simulink model "simulink_control"  (R2025b)
settings: Solver=ode4  StartTime=0.0  StopTime=inf  FixedStep=0.016  RelTol=1e-3
values from neighbouring files (symbols this model uses):
  accelerometer_sensor = wb_robot_get_device('accelerometer')    [simulink_control_app.m]
  alpha_pitch = 0.85    [simulink_control_app.m]
  gps_sensor = wb_robot_get_device('gps')    [simulink_control_app.m]
  gyro_sensor = wb_robot_get_device('gyro')    [simulink_control_app.m]
  inertial_unit = wb_robot_get_device('inertial_unit')    [simulink_control_app.m]
  left_trushter_motor = wb_robot_get_device('left_motor')    [simulink_control_app.m]
  right_trushter_motor = wb_robot_get_device('right_motor')    [simulink_control_app.m]
  TIME_STEP = 16    [simulink_control_app.m]
undefined symbols (not defined in the file or in its folder): gray, mission_waypoints
libraries: simulink_extras x5, eeGeneralControl x2
settings Model: Creator=Harun  LastModifiedBy=Szymon
settings DebuggingCC: UnderSpecifiedDimensionMsg=warning

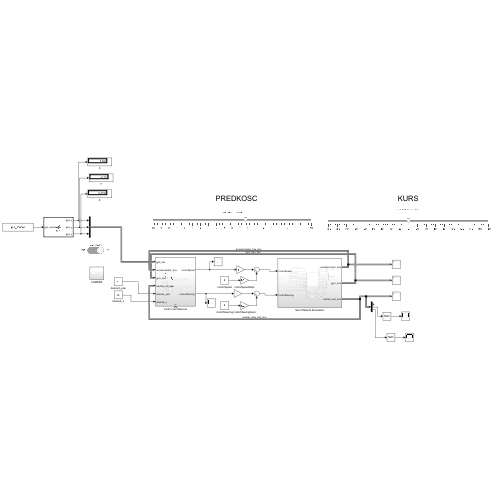
[thumbnail: Simulink's stored preview of the top-level diagram]
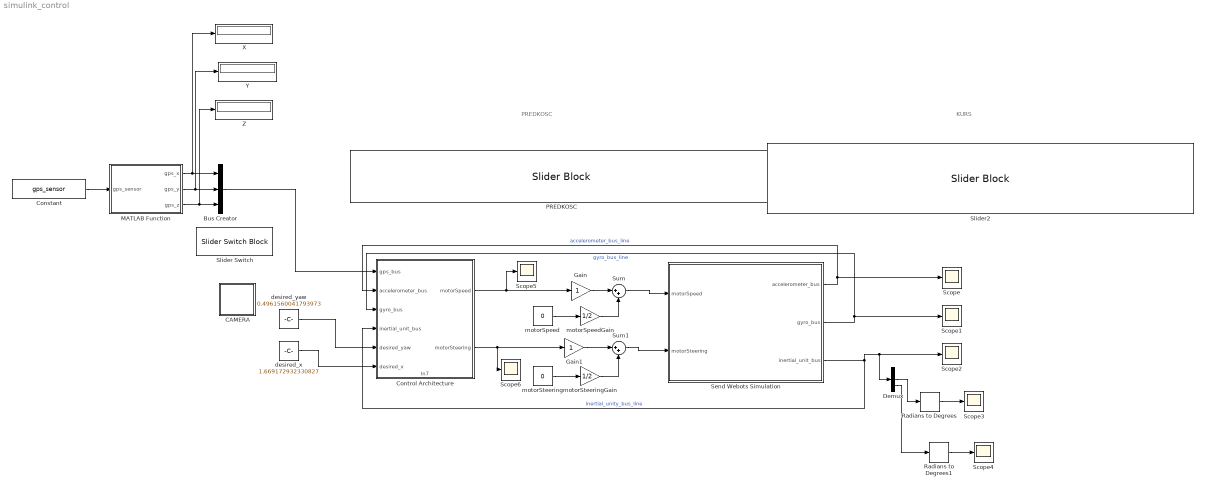
== system simulink_control ==
  note: KURS
  note: PREDKOSC
  Bus Creator : BusCreator  Inputs=3
  CAMERA : Subsystem
  Constant : Constant  Value=gps_sensor
  Control Architecture : Subsystem
      settings: PortSchema="{\"entries\":[{\"content\":{\"sides\":[{\"content\":{\"connectorIds\":[\"In1\",\"In2\",\"In3\",\"In4\",\"In5\",\"In6\"]},\"type\":\"ConnectorPlacement.EquallySpacedRectSide\",\"uuid\":\"94cabca2-e76e-4691-9816-b95fb886a2a7\"},{\"content\":{\"connectorIds\":[\"Out1\",\"Out2\"],\"side\":\"RIGHT\"},\"type\":\"ConnectorPlacement.EquallySpacedRectSide\",\"uuid\":\"240d2e1d-620c-4ca0-9643-bfc077ee6341\"},{\"content\":{\"side\":\"TOP\"},\"type\":\"ConnectorPlacement.EquallySpacedRectSide\",\"uuid\":\"858b813a-0718-4a6f-97d6-2c7be5dc6086\"},{\"content\":{\"connectorIds\":[\"In7\"],\"side\":\"BOTTOM\"},\"type\":\"ConnectorPlacement.EquallySpacedRectSide\",\"uuid\":\"e25d5035-11e6-4256-b3cd-0a1c699f2cde\"}]},\"type\":\"ConnectorPlacement.EquallySpacedConnector\",\"uuid\":\"155b933b-e855-4e90-a0aa-f79b0a1ce075\"}],\"packageUris\":[\"http://schema.mathworks.com/mf0/Connector/R2020b\"],\"version\":\"1.0\"}"
  Demux : Demux  Outputs=3
  Gain : Gain
  Gain1 : Gain
  MATLAB Function : MATLAB Function  TreatAsAtomicUnit=on
  PREDKOSC : SliderBlock  ScaleMin=-10  ScaleMax=10
  Radians to Degrees : simulink_extras/Transformations/Radians to Degrees
  Radians to Degrees1 : simulink_extras/Transformations/Radians to Degrees
  Scope{,1..6} (7 alike) : Scope
      Scope settings: ActiveDisplayYMinimum=-30.6391  ActiveDisplayYMaximum=29.79687
      Scope1 settings: ActiveDisplayYMinimum=-12220.56497  ActiveDisplayYMaximum=12217.33322
      Scope2 settings: ActiveDisplayYMinimum=-3.8392  ActiveDisplayYMaximum=3.73806
      Scope3 settings: ActiveDisplayYMinimum=-1.49091  ActiveDisplayYMaximum=-1.14094  DataLoggingVariableName=ScopeData2
      Scope4 settings: ActiveDisplayYMinimum=-48.59786  ActiveDisplayYMaximum=-34.20452  DataLoggingVariableName=ScopeData2
      Scope5 settings: ActiveDisplayYMinimum=-0.00358  ActiveDisplayYMaximum=0.03222  DataLoggingVariableName=ScopeData5
      Scope6 settings: ActiveDisplayYMinimum=-0.15563  ActiveDisplayYMaximum=1.4007  DataLoggingVariableName=ScopeData2
  Send Webots Simulation : Subsystem
  Slider Switch : SliderSwitchBlock
  Slider2 : SliderBlock  ScaleMin=-180  ScaleMax=180  TickInterval=20
  Sum : Sum  Inputs=|++
  Sum1 : Sum  Inputs=|++
  X : Display
  Y : Display
  Z : Display
  desired_x : Constant  Value=1.669172932330827
  desired_yaw : Constant  Value=0.4961560041793973
  motorSpeed : Constant  Value=0
  motorSpeedGain : Gain  Gain=1/2
  motorSteering : Constant  Value=0
  motorSteeringGain : Gain  Gain=1/2
  wires:
  motorSteering/1 -> motorSteeringGain/1
  motorSpeed/1 -> motorSpeedGain/1
  Sum/1 -> Send Webots Simulation/1(motorSpeed)
  Control Architecture/1(motorSpeed) -> Scope5/1, Gain/1
  Control Architecture/2(motorSteering) -> Scope6/1, Gain1/1
  Sum1/1 -> Send Webots Simulation/2(motorSteering)
  motorSpeedGain/1 -> Sum/2
  motorSteeringGain/1 -> Sum1/2
  Send Webots Simulation/1(accelerometer_bus) -> Control Architecture/2(accelerometer_bus), Scope/1  "accelerometer_bus_line"
  Send Webots Simulation/2(gyro_bus) -> Control Architecture/3(gyro_bus), Scope1/1  "gyro_bus_line"
  Send Webots Simulation/3(inertial_unit_bus) -> Demux/1, Scope2/1, Control Architecture/4(inertial_unit_bus)  "inertial_unity_bus_line"
  Gain/1 -> Sum/1
  Demux/2 -> Radians to Degrees/1
  Radians to Degrees/1 -> Scope3/1
  Radians to Degrees1/1 -> Scope4/1
  Demux/3 -> Radians to Degrees1/1
  Gain1/1 -> Sum1/1
  desired_x/1 -> Control Architecture/6(desired_x)
  desired_yaw/1 -> Control Architecture/5(desired_yaw)
  Constant/1 -> MATLAB Function/1(gps_sensor)
  MATLAB Function/2(gps_y) -> Y/1, Bus Creator/2
  MATLAB Function/3(gps_z) -> Z/1, Bus Creator/3
  MATLAB Function/1(gps_x) -> X/1, Bus Creator/1
  Bus Creator/1 -> Control Architecture/1(gps_bus)

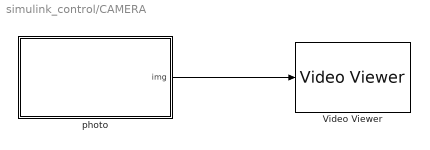
== system simulink_control/CAMERA ==
  Video Viewer : VideoViewer  colormapValue=gray(256)  FigPos=[1 1158 1920 1061]
  photo : MATLAB Function  TreatAsAtomicUnit=on
  wires:
  photo/1(img) -> Video Viewer/1

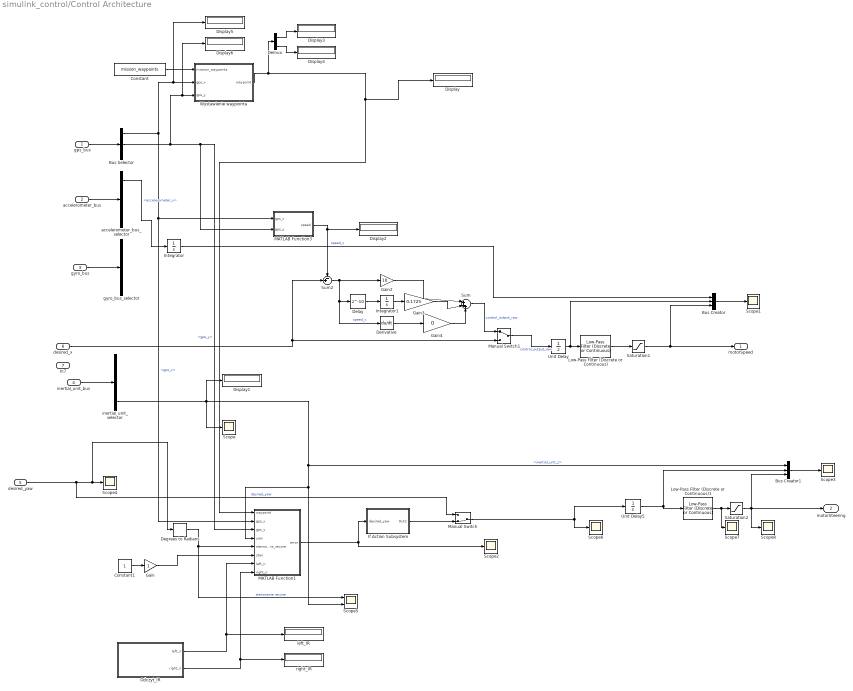
== system simulink_control/Control Architecture ==
  gps_bus : Inport
  accelerometer_bus : Inport  Port=2
  gyro_bus : Inport  Port=3
  inertial_unit_bus : Inport  Port=4
  desired_yaw : Inport  Port=5
  desired_x : Inport  Port=6
  In7 : Inport  Port=7
  Bus Creator : BusCreator  Inputs=3
  Bus Creator1 : BusCreator  Inputs=3
  Bus Selector : BusSelector  OutputSignals=gps_x,gps_y,gps_z
  Constant : Constant  Value=mission_waypoints
  Constant1 : Constant
  Degrees to Radians : simulink_extras/Transformations/Degrees to Radians
  Delay : Delay  DelayLength=10
  Demux : Demux  Outputs=2
  Derivative : Derivative  CoefficientInTFapproximation=0.016
  Display{,1..6} (7 alike) : Display
  Gain : Gain
  Gain2 : Gain  Gain=10
  Gain3 : Gain  Gain=0.1725
  Gain4 : Gain  Gain=0
  If Action Subsystem : Subsystem  TreatAsAtomicUnit=on
  Integrator : Integrator
  Integrator1 : Integrator
  Low-Pass Filter (Discrete or Continuous) : eeGeneralControl/Low-Pass Filter (Discrete or Continuous)  K=1  T=0.016  B=inf  A=-inf  init_option=Inherited from block input  x0=0  Ts=-1
  Low-Pass Filter (Discrete or Continuous)1 : eeGeneralControl/Low-Pass Filter (Discrete or Continuous)  K=1  T=0.016  B=inf  A=-inf  init_option=Inherited from block input  x0=0  Ts=-1
  MATLAB Function1 : MATLAB Function  TreatAsAtomicUnit=on
  MATLAB Function3 : MATLAB Function  TreatAsAtomicUnit=on
  Manual Switch : ManualSwitch  CurrentSetting=0
  Manual Switch1 : ManualSwitch
  Odczyt_IR : MATLAB Function  TreatAsAtomicUnit=on
  Saturation1 : Saturate  UpperLimit=15  LowerLimit=-15
  Saturation2 : Saturate  UpperLimit=5  LowerLimit=-5
  Scope{,1..4,6..8} (8 alike) : Scope
      Scope settings: ActiveDisplayYMinimum=-0.84582  ActiveDisplayYMaximum=3.34904
      Scope1 settings: ActiveDisplayYMinimum=-78.38231  ActiveDisplayYMaximum=106.01245  DataLoggingVariableName=ScopeData2
      Scope2 settings: ActiveDisplayYMinimum=-0.00316  ActiveDisplayYMaximum=0.00341  DataLoggingVariableName=ScopeData3
      Scope3 settings: ActiveDisplayYMinimum=-48028.32937  ActiveDisplayYMaximum=47920.10481
      Scope4 settings: ActiveDisplayYMinimum=85.82399  ActiveDisplayYMaximum=105.82399
      Scope6 settings: ActiveDisplayYMinimum=-1006.23593  ActiveDisplayYMaximum=1051.55838  DataLoggingVariableName=ScopeData3
      Scope7 settings: ActiveDisplayYMinimum=-7.95026  ActiveDisplayYMaximum=65.1796  DataLoggingVariableName=ScopeData4
      Scope8 settings: ActiveDisplayYMinimum=-0.15563  ActiveDisplayYMaximum=1.4007  DataLoggingVariableName=ScopeData5
  Scope5 : Scope  NumInputPorts=2
      settings: ActiveDisplayYMinimum=-3.49256  ActiveDisplayYMaximum=3.48254  DataLoggingVariableName=ScopeData2
  Sum : Sum  Inputs=|+++
  Sum2 : Sum  Inputs=-+|
  Unit Delay : UnitDelay  SampleTime=-1  HasFrameUpgradeWarning=on
  Unit Delay5 : UnitDelay  SampleTime=-1  HasFrameUpgradeWarning=on
  Wystawienie waypointa : MATLAB Function  TreatAsAtomicUnit=on
  accelerometer_bus_selector : BusSelector  OutputSignals=accelerometer_x,accelerometer_y,accelerometer_z
  gyro_bus_selector : BusSelector  OutputSignals=gyro_x,gyro_y,gyro_z
  inertial_unit_selector : BusSelector  OutputSignals=inertial_unit_x,inertial_unit_y,inertial_unit_z
  left_IR : Display
  right_IR : Display
  motorSpeed : Outport
  motorSteering : Outport  Port=2
  wires:
  accelerometer_bus/1 -> accelerometer_bus_selector/1
  gyro_bus/1 -> gyro_bus_selector/1
  inertial_unit_bus/1 -> inertial_unit_selector/1
  Bus Creator/1 -> Scope1/1
  inertial_unit_selector/3 -> Scope/1, Display1/1, Scope5/2, MATLAB Function1/4(yaw), Bus Creator1/1  "<inertial_unit_z>"
  Saturation1/1 -> motorSpeed/1, Bus Creator/3
  Integrator/1 -> Bus Creator/1  "speed_x"
  Unit Delay/1 -> Bus Creator/2, Low-Pass Filter (Discrete or Continuous)/1
  Low-Pass Filter (Discrete or Continuous)/1 -> Saturation1/1
  Unit Delay5/1 -> Low-Pass Filter (Discrete or Continuous)1/1, Bus Creator1/2
  Bus Creator1/1 -> Scope3/1
  accelerometer_bus_selector/1 -> Integrator/1  "<accelerometer_x>"
  gps_bus/1 -> Bus Selector/1
  Bus Selector/1 -> MATLAB Function1/2(gps_x), MATLAB Function3/1(gps_x), Display5/1, Wystawienie waypointa/2(gps_x)  "<gps_x>"
  Bus Selector/2 -> MATLAB Function3/2(gps_y), MATLAB Function1/3(gps_y), Display6/1, Wystawienie waypointa/3(gps_y)  "<gps_y>"
  Manual Switch/1 -> Unit Delay5/1, Scope6/1
  desired_yaw/1 -> Manual Switch/1, Scope4/1, Degrees to Radians/1  "desired_yaw"
  Saturation2/1 -> Scope8/1, motorSteering/1, Bus Creator1/3
  Degrees to Radians/1 -> Scope5/1, MATLAB Function1/5(sterwowanie_reczne)  "sterowanie reczne"
  Low-Pass Filter (Discrete or Continuous)1/1 -> Scope7/1, Saturation2/1
  Wystawienie waypointa/1(waypoint) -> MATLAB Function1/1(waypoint), Display/1, Demux/1
  MATLAB Function3/1(speed) -> Sum2/1, Display2/1
  desired_x/1 -> Sum2/2, Manual Switch1/2
  Sum2/1 -> Gain2/1, Derivative/1, Delay/1  "speed_x"
  Manual Switch1/1 -> Unit Delay/1  "control_output_raw"
  Integrator1/1 -> Gain3/1
  Gain3/1 -> Sum/2
  Gain2/1 -> Sum/1
  Derivative/1 -> Gain4/1
  Gain4/1 -> Sum/3
  Sum/1 -> Manual Switch1/1  "control_output_raw"
  MATLAB Function1/1(error) -> Scope2/1, If Action Subsystem/1(desired_yaw)
  If Action Subsystem/1(Out2) -> Manual Switch/2
  Delay/1 -> Integrator1/1
  Demux/1 -> Display3/1
  Demux/2 -> Display4/1
  Constant/1 -> Wystawienie waypointa/1(mission_waypoints)
  Gain/1 -> MATLAB Function1/6(stan)
  Constant1/1 -> Gain/1
  Odczyt_IR/1(left_ir) -> MATLAB Function1/7(left_ir), left_IR/1
  Odczyt_IR/2(right_ir) -> MATLAB Function1/8(right_ir), right_IR/1

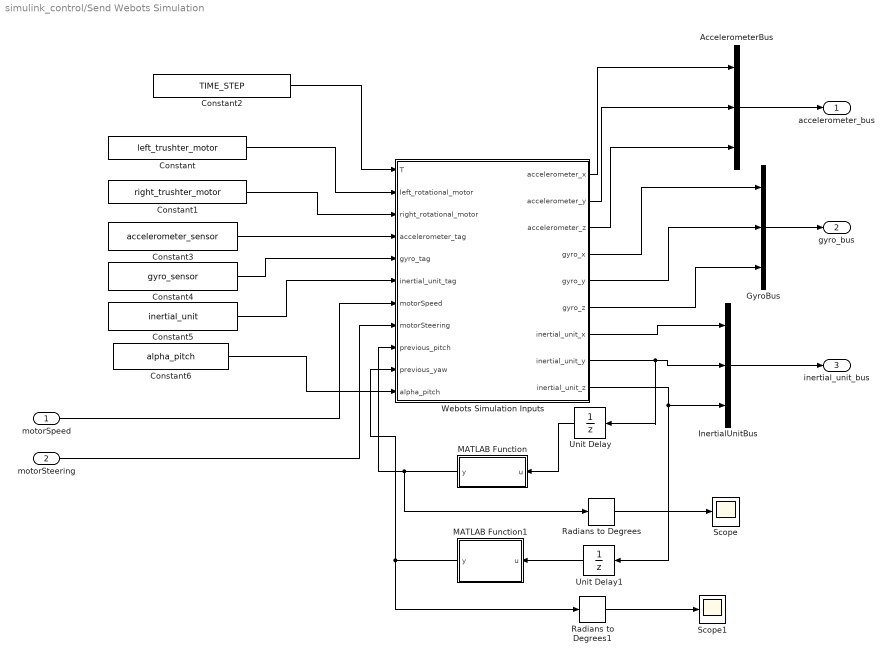
== system simulink_control/Send Webots Simulation ==
  motorSpeed : Inport
  motorSteering : Inport  Port=2
  AccelerometerBus : BusCreator  Inputs=3
  Constant : Constant  Value=left_trushter_motor
  Constant1 : Constant  Value=right_trushter_motor
  Constant2 : Constant  Value=TIME_STEP
  Constant3 : Constant  Value=accelerometer_sensor
  Constant4 : Constant  Value=gyro_sensor
  Constant5 : Constant  Value=inertial_unit
  Constant6 : Constant  Value=alpha_pitch
  GyroBus : BusCreator  Inputs=3
  InertialUnitBus : BusCreator  Inputs=3
  MATLAB Function : MATLAB Function  TreatAsAtomicUnit=on
  MATLAB Function1 : MATLAB Function  TreatAsAtomicUnit=on
  Radians to Degrees : simulink_extras/Transformations/Radians to Degrees
  Radians to Degrees1 : simulink_extras/Transformations/Radians to Degrees
  Scope : Scope
      settings: ActiveDisplayYMinimum=-1.32337  ActiveDisplayYMaximum=0.14704
  Scope1 : Scope
      settings: ActiveDisplayYMinimum=-221.28069  ActiveDisplayYMaximum=223.17839  DataLoggingVariableName=ScopeData3
  Unit Delay : UnitDelay  SampleTime=-1  HasFrameUpgradeWarning=on
  Unit Delay1 : UnitDelay  SampleTime=-1  HasFrameUpgradeWarning=on
  Webots Simulation Inputs : MATLAB Function  TreatAsAtomicUnit=on
  accelerometer_bus : Outport
  gyro_bus : Outport  Port=2
  inertial_unit_bus : Outport  Port=3
  wires:
  motorSpeed/1 -> Webots Simulation Inputs/7(motorSpeed)
  Constant1/1 -> Webots Simulation Inputs/3(right_rotational_motor)
  Constant2/1 -> Webots Simulation Inputs/1(T)
  Constant/1 -> Webots Simulation Inputs/2(left_rotational_motor)
  Webots Simulation Inputs/2(accelerometer_y) -> AccelerometerBus/2
  Webots Simulation Inputs/1(accelerometer_x) -> AccelerometerBus/1
  Webots Simulation Inputs/3(accelerometer_z) -> AccelerometerBus/3
  AccelerometerBus/1 -> accelerometer_bus/1
  Constant3/1 -> Webots Simulation Inputs/4(accelerometer_tag)
  motorSteering/1 -> Webots Simulation Inputs/8(motorSteering)
  Constant4/1 -> Webots Simulation Inputs/5(gyro_tag)
  Webots Simulation Inputs/6(gyro_z) -> GyroBus/3
  Webots Simulation Inputs/5(gyro_y) -> GyroBus/2
  GyroBus/1 -> gyro_bus/1
  Webots Simulation Inputs/4(gyro_x) -> GyroBus/1
  Webots Simulation Inputs/7(inertial_unit_x) -> InertialUnitBus/1
  Webots Simulation Inputs/8(inertial_unit_y) -> Unit Delay/1, InertialUnitBus/2
  Webots Simulation Inputs/9(inertial_unit_z) -> Unit Delay1/1, InertialUnitBus/3
  InertialUnitBus/1 -> inertial_unit_bus/1
  Constant5/1 -> Webots Simulation Inputs/6(inertial_unit_tag)
  Constant6/1 -> Webots Simulation Inputs/11(alpha_pitch)
  MATLAB Function/1(y) -> Radians to Degrees/1, Webots Simulation Inputs/9(previous_pitch)
  Unit Delay/1 -> MATLAB Function/1(u)
  Radians to Degrees/1 -> Scope/1
  Unit Delay1/1 -> MATLAB Function1/1(u)
  Radians to Degrees1/1 -> Scope1/1
  MATLAB Function1/1(y) -> Radians to Degrees1/1, Webots Simulation Inputs/10(previous_yaw)

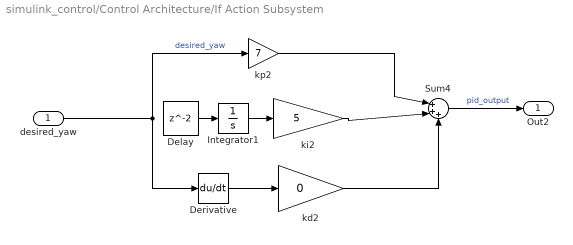
== system simulink_control/Control Architecture/If Action Subsystem ==
  desired_yaw : Inport
  Delay : Delay
  Derivative : Derivative
  Integrator1 : Integrator
  Sum4 : Sum  Inputs=|+++
  kd2 : Gain  Gain=0
  ki2 : Gain  Gain=5
  kp2 : Gain  Gain=7
  Out2 : Outport
  wires:
  Sum4/1 -> Out2/1  "pid_output"
  kp2/1 -> Sum4/1
  ki2/1 -> Sum4/2
  Integrator1/1 -> ki2/1
  desired_yaw/1 -> Derivative/1, kp2/1  "desired_yaw"
  kd2/1 -> Sum4/3
  Derivative/1 -> kd2/1
  Delay/1 -> Integrator1/1

== matlab function simulink_control/Control Architecture/MATLAB Function1 ==
  data: waypoint input; error output; gps_x input; gps_y input; yaw input; sterwowanie_reczne input; stan input; left_ir input; right_ir input
function error = guidance(waypoint, gps_x, gps_y, yaw, sterwowanie_reczne, stan, left_ir, right_ir)
persistent timer_ucieczki kat_ucieczki

if isempty(timer_ucieczki)
    timer_ucieczki = 0;
    kat_ucieczki = 0;
end

if stan == 1
    % 1. KURS DO WAYPOINTA
    dx = waypoint(1) - gps_x;
    dy = waypoint(2) - gps_y;
    psi_nav = atan2(dx, dy);      
    
    % 2. PARAMETRY LASERÓW (Zasięg twardy: 5 metrów)
    % Przy tabeli [0 0 0, 5 1000 0] wartość 950 oznacza reakcję z 4.75 metra.
    % Laser uderza w beczkę -> natychmiastowa reakcja!
    threshold = 950;       
    
    % Czas ucieczki musi być długi (np. 300), bo statek po ostrym skręcie 
    % szybko straci beczkę z "pola widzenia" krótkiego lasera. 
    % Ten czas pozwala mu odpłynąć na bok, by nie zahaczyć tyłem (rufą).
    czas_ucieczki = 200;   
    
    % 3. LOGIKA OMIJANIA (ZATRZASK)
    if left_ir < threshold || right_ir < threshold
        
        % ZATRZASK: Gwałtowna decyzja w ułamku sekundy
        if timer_ucieczki == 0
            if left_ir <= right_ir
                kat_ucieczki = pi/2.5;  % Ekstremalny unik w prawo (72 stopnie)
            else
                kat_ucieczki = -pi/2.5; % Ekstremalny unik w lewo (72 stopnie)
            end
        end
        
        % Dopóki laser widzi beczkę w promieniu 5m, trzymaj timer na maksa
        timer_ucieczki = czas_ucieczki;
    end
    
    % 4. MIKSER SYGNAŁÓW
    if timer_ucieczki > 0
        psi = psi_nav + kat_ucieczki;
        timer_ucieczki = timer_ucieczki - 1; 
    else
        psi = psi_nav;
    end
    
    % MATEMATYKA KĄTÓW
    psi = mod(psi, 2*pi); 
    heading = pi/2 - yaw;
    heading = mod(heading, 2*pi);
    error = atan2(sin(psi - heading), cos(psi - heading));
else
    % TRYB MANUALNY
    error = sterwowanie_reczne - yaw;
    error = -atan2(sin(error), cos(error));
end
end

== matlab function simulink_control/Control Architecture/MATLAB Function3 ==
  data: gps_x input; speed output; gps_y input
function speed = fcn(gps_x, gps_y)

persistent previous_x previous_y

time = 0.016;

if isempty(previous_x)
    previous_x = gps_x;
    previous_y = gps_y;
end

dx = gps_x - previous_x;
dy = gps_y - previous_y;

speed = sqrt(dx^2 + dy^2) / time;

previous_x = gps_x;
previous_y = gps_y;

end

== matlab function simulink_control/Send Webots Simulation/MATLAB Function1 ==
  data: u input; y output
function y = fcn(u)

y = u;

== matlab function simulink_control/MATLAB Function ==
  data: gps_sensor input; gps_x output; gps_y output; gps_z output
function [gps_x, gps_y, gps_z] = fcn(gps_sensor)

coder.extrinsic('wb_gps_get_values');


gps_x = 0;
gps_y = 0;
gps_z = 0;

position=wb_gps_get_values(gps_sensor);

gps_x=position(1);
gps_y=position(2);
gps_z=position(3);

== matlab function simulink_control/Send Webots Simulation/Webots Simulation Inputs ==
  data: T input; left_rotational_motor input; right_rotational_motor input; accelerometer_tag input; gyro_tag input; inertial_unit_tag input; motorSpeed input; accelerometer_x output; accelerometer_y output; accelerometer_z output; motorSteering input; gyro_x output; gyro_y output; gyro_z output; inertial_unit_x output; inertial_unit_y output; inertial_unit_z output; previous_pitch input; previous_yaw input; alpha_pitch input
function [accelerometer_x,accelerometer_y,accelerometer_z,gyro_x,gyro_y,gyro_z,inertial_unit_x,inertial_unit_y,inertial_unit_z] = simulation(T,left_rotational_motor,right_rotational_motor,accelerometer_tag,gyro_tag,inertial_unit_tag ...
    ,motorSpeed,motorSteering,previous_pitch,previous_yaw,alpha_pitch)

accelerometer_x = 0.0;
accelerometer_y = 0.0;
accelerometer_z = 0.0;

gyro_x=0.0;
gyro_y=0.0;
gyro_z=0.0;


wb_robot_step(T)
wb_motor_set_position(left_rotational_motor, Inf);
wb_motor_set_position(right_rotational_motor, Inf);
wb_motor_set_velocity(right_rotational_motor, motorSpeed-motorSteering);
wb_motor_set_velocity(left_rotational_motor, motorSpeed+motorSteering);

%period = wb_accelerometer_get_sampling_period(accelerometer_tag)
accelerometer_values = zeros(1, 3); 
accelerometer_values = wb_accelerometer_get_values(accelerometer_tag);
accelerometer_x = accelerometer_values(1);
accelerometer_y = accelerometer_values(2);
accelerometer_z = accelerometer_values(3);



gyro_values = zeros(1, 3); 
gyro_values = wb_gyro_get_values(gyro_tag);

gyro_x = gyro_values(1);
gyro_y = gyro_values(2);
gyro_z = gyro_values(3);


inertial_unit_values = zeros(1, 3); 
inertial_unit_values = wb_inertial_unit_get_roll_pitch_yaw(inertial_unit_tag);



inertial_unit_x = inertial_unit_values(1);
inertial_unit_y = inertial_unit_values(2);
inertial_unit_z = inertial_unit_values(3);

interial_unit_y=alpha_pitch*inertial_unit_y+(1-alpha_pitch)*previous_pitch;

inertial_unit_z=alpha_pitch*inertial_unit_z+(1-alpha_pitch)*previous_yaw;


end

== matlab function simulink_control/Control Architecture/Wystawienie waypointa ==
  data: mission_waypoints input; waypoint output; gps_x input; gps_y input
function waypoint = fcn(mission_waypoints, gps_x, gps_y)
    % persistent pamięta wartość pomiędzy klatkami symulacji
    persistent wp_idx
    
    % Inicjalizacja TYLKO przy starcie
    if isempty(wp_idx)
        wp_idx = 1;
    end
    
    % Sprawdzenie, ile punktów ma misja
    num_wps = size(mission_waypoints, 1);
    
    % Zabezpieczenie przed wyjściem poza tablicę
    if wp_idx > num_wps
        wp_idx = 1;
    end
    
    % Odczytanie współrzędnych aktualnego celu
    target_x = mission_waypoints(wp_idx, 1);
    target_y = mission_waypoints(wp_idx, 2);
    
    % Obliczenie dystansu drona do aktualnego celu
    dist = sqrt((target_x - gps_x)^2 + (target_y - gps_y)^2);
    
    % PROMIEŃ ZALICZENIA (2 metry)
    if dist < 2.0
        wp_idx = wp_idx + 1;
        
        % KLUCZOWA ZMIANA: ZAPĘTLENIE TRASY
        % Jeśli osiągnęliśmy ostatni punkt, wracamy do pierwszego!
        if wp_idx > num_wps
            wp_idx = 1;
        end
    end
    
    % Zwrócenie gotowego waypointa 
    waypoint = [mission_waypoints(wp_idx, 1); mission_waypoints(wp_idx, 2)];
end

== matlab function simulink_control/Control Architecture/Odczyt_IR ==
  data: left_ir output; right_ir output
function [left_ir, right_ir] = read_sensors()
    coder.extrinsic('wb_robot_get_device', 'wb_distance_sensor_get_value');
    left_ir = 0.0;
    right_ir = 0.0;
    tag_left = wb_robot_get_device('left_ir');
    tag_right = wb_robot_get_device('right_ir');
    left_ir = wb_distance_sensor_get_value(tag_left);
    right_ir = wb_distance_sensor_get_value(tag_right);
end

== matlab function simulink_control/Send Webots Simulation/MATLAB Function ==
  data: u input; y output
function y = fcn(u)

y = u;

== matlab function simulink_control/CAMERA/photo ==
  data: img output
function img = photo
    % Deklarujemy nasz nowy, bezpieczny skrypt
    coder.extrinsic('wb_robot_get_device', 'get_camera_safe');
    
    % Inicjalizacja wyjścia
    img = zeros(240, 320, 3, 'uint8');
    
    % Pobranie uchwytu do kamery
    camera = 0; 
    camera = wb_robot_get_device('camera');
    
    % Pobranie obrazu przez naszą bezpieczną tarczę
    if camera > 0
        img = get_camera_safe(camera);
    end
end
